simulink model "PDCb1"  (R2017a)
settings: Solver=VariableStepAuto  StartTime=0.0  StopTime=6000  RelTol=1e-3
values from neighbouring files (symbols this model uses):
  A = [-0.003401570000000  -0.000000016230000 ... (first row only)    [Lyglobal.m]
  A1 = [-0.002786000000000  -0.000000019880000 ... (first row only)    [Lyglobal.m]
  B = [1;0]    [Lyglobal.m]
  B1 = [1;0]    [Lyglobal.m]
  C = [1 0]    [Lyglobal.m]
  C1 = [1 0]    [Lyglobal.m]
  D = 0    [Lyglobal.m]
  D1 = 0    [Lyglobal.m]
  K = [8.997598430000000   0.008999983770000]    [Lyglobal.m]    (also in PDCtracking.m = [K k]; planta.m = acker(A,B,P))
  K1 = [7.997223999999999   0.000079980120000]    [Lyglobal.m]    (also in Planta100.m = acker(A1,B1,P))
libraries: fuzblock x4
settings Model: Creator=Dell  LastModifiedBy=Dell

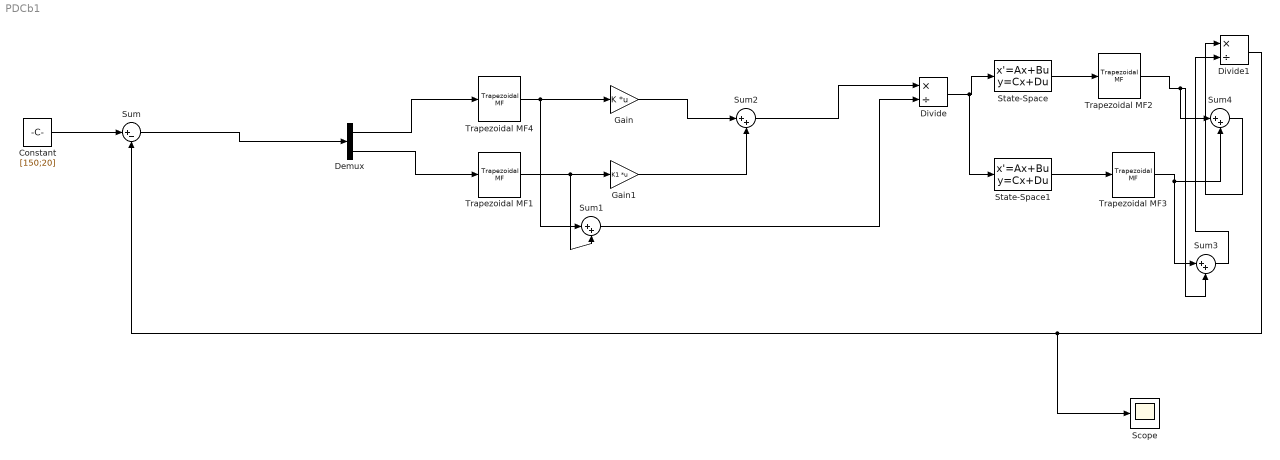
== system PDCb1 ==
  Constant : Constant  Value=[150;20]  VectorParams1D=off
  Demux : Demux  Outputs=2
  Divide : Product  Inputs=*/
  Divide1 : Product  Inputs=*/
  Gain : Gain  Gain=K  Multiplication=Matrix(K*u)
  Gain1 : Gain  Gain=K1  Multiplication=Matrix(K*u)
  Scope : Scope
  State-Space : StateSpace  A=A  B=B  C=C  D=D  X0=0
  State-Space1 : StateSpace  A=A1  B=B1  C=C1  D=D1  X0=0
  Sum : Sum  Inputs=|+-
  Sum{1..4} (4 alike) : Sum  Inputs=|++
  Trapezoidal MF1 : fuzblock/Membership  Functions/Trapezoidal MF  a=101  b=125  c=150  d=200
      settings: SourceProductName=Fuzzy Logic Toolbox  SourceProductBaseCode=FL
  Trapezoidal MF2 : fuzblock/Membership  Functions/Trapezoidal MF  a=0  b=45  c=90  d=135
      settings: SourceProductName=Fuzzy Logic Toolbox  SourceProductBaseCode=FL
  Trapezoidal MF3 : fuzblock/Membership  Functions/Trapezoidal MF  a=180  b=180+45  c=270  d=360
      settings: SourceProductName=Fuzzy Logic Toolbox  SourceProductBaseCode=FL
  Trapezoidal MF4 : fuzblock/Membership  Functions/Trapezoidal MF  a=1  b=50  c=75  d=100
      settings: SourceProductName=Fuzzy Logic Toolbox  SourceProductBaseCode=FL
  wires:
  Constant/1 -> Sum/1
  Demux/1 -> Trapezoidal MF4/1
  Demux/2 -> Trapezoidal MF1/1
  Sum/1 -> Demux/1
  Trapezoidal MF4/1 -> Sum1/1, Gain/1
  Trapezoidal MF1/1 -> Sum1/2, Gain1/1
  Sum2/1 -> Divide/1
  Sum1/1 -> Divide/2
  Gain/1 -> Sum2/1
  Gain1/1 -> Sum2/2
  Divide/1 -> State-Space1/1, State-Space/1
  State-Space/1 -> Trapezoidal MF2/1
  State-Space1/1 -> Trapezoidal MF3/1
  Trapezoidal MF3/1 -> Sum4/2, Sum3/1
  Trapezoidal MF2/1 -> Sum4/1, Sum3/2
  Sum4/1 -> Divide1/1
  Sum3/1 -> Divide1/2
  Divide1/1 -> Scope/1, Sum/2
